simulink model "PubIfDecisionTOS_MDL"  (R2020b)
settings: configuration reference "DspaceConfig" (kept outside this file)
PostLoadFcn:
  | if any(exist('dsrtsu_mdlpostloadfcn', 'file') ~= 0), dsrtsu_mdlpostloadfcn('Execute', bdroot); end
InitFcn:
  | , if any(exist('dsmpb_private', 'file') ~= 0), dsmpb_private('dsmpb_mdlclblib', 'Init', bdroot); end,
undefined symbols (not defined in the file or in its folder): C_TOS_ACCEgoRAxletoFbumplength_m, C_TOS_ACCTargetFront_Flag, C_TOS_AEBJAPedObjDxThre_Val, C_TOS_AEBJAPedObjDyThre_Val, C_TOS_AEBJATargetSize_Val, C_TOS_AEBJAVehObjDxThre_Val, C_TOS_AEBJAVehObjDyThre_Val, C_TOS_AEBJuncPedTargetSize_Val, C_TOS_AEBLatObjDxThre_Val, C_TOS_AEBLatPedDyThre_Val, C_TOS_AEBLatTargetSize_Val, C_TOS_AEBLongTargetInEgoFront_Flag, C_TOS_axAbsGround_Parameter, C_TOS_CameraConfirmedFlag, C_TOS_CNsubjWidth, C_TOS_CurrentLaneCoreMinWidth_Val, C_TOS_CutInProb_Val_Zero, C_TOS_CutOutProb_Val_Zero, C_TOS_D2R_Val, C_TOS_DefaultValueObjectToCenterLine_dy, C_TOS_EgoCarWidth_Val, C_TOS_EgoDxRefPoint_m, C_TOS_EgoRAxletoFbumplength_m, C_TOS_HalfWidthVehicle_Con, C_TOS_HWA_CurrentLaneFlag, C_TOS_HWA_LeftLaneFlag, C_TOS_HWA_MovingDir_Vaild, C_TOS_HWA_MovState_Vaild, C_TOS_HWA_RightLaneFlag, C_TOS_LaneLineCourseErrorFront, C_TOS_LaneLineCourseErrorRear, C_TOS_MotorbikeDefaultWidth_m, C_TOS_NumberOfEffectiveTargets, C_TOS_Obj_Age_Val, C_TOS_Objdx_Constraint_Val, C_TOS_ObjectDefaultWidth_m, C_TOS_ObjInCurrentLane_Val, C_TOS_ObjInCurrentLaneValid, C_TOS_ObjInLeftLaneValid, C_TOS_ObjInRightLaneValid, C_TOS_ObjNotInCurrentLane_Val, C_TOS_ObjNotREElementType, C_TOS_ObjPredictDis_dy_ConstantVal_Zeros, C_TOS_ObjToCenterLine_ConstantVal_Zeros, C_TOS_OFMObjIDInvilad_Val, C_TOS_PIL_LatDisCons_Val_zero, C_TOS_PIL_ObjectCutInFlag_b, C_TOS_PIL_ObjectCutOutFlag_b, C_TOS_PIL_ObjLaneProb_al_Val, C_TOS_PP_ObjFusType_FC_Confirm_b, C_TOS_PP_ObjFusType_FC_FR_Confirm_b, C_TOS_PP_ObjFusType_FR_Confirm_b, C_TOS_RE_80BoolDefault_Val, C_TOS_RE_80Single181Default_Val, C_TOS_RE_80Single255Default_Val, C_TOS_RE_80Uint8Default_Val, C_TOS_RE_D2R, C_TOS_RE_D_180_Val, C_TOS_RE_InvalidObjectID_Val, C_TOS_RE_InvalidTargetChainDir_Val ... (+142)
libraries: simulink x1650, TOS_LIB x361, canfdmsglib x14
(part 64 of 69)

== stateflow chart PubIfDecisionTOS_MDL/TOS_20201112/TOS_2012080320/TOS/ACC/TOS_ACCLeftLane/ACC_LeftLane_Target/TOS_ACC_P2/ACC_P2_Targe/ACC_P2_Targe/TOS_ACC_FusionTypeConfirm/Subsystem1/TOS_ObjMovStateCfmFlow1 ==
  note: TOS_ObjMovStateCfm Coding:
      | 0: Object default moving state
      | 1：Object had been moving
      | 2: Object is moving
  (default) -> (junction 1)
  (junction 1) -> (junction 3) [order 1] : [Target_ID_K1 ~=C_TOS_OFMObjIDInvilad_Val&&...
      | Target_ID_K2 ~= C_TOS_OFMObjIDInvilad_Val]
  (junction 1) -> (junction 38) [order 2] : {
      |   TOS_ObjMovStateCfm = uint8(0);
      | }
  (junction 3) -> (junction 5)
  (junction 5) -> (junction 7) [order 1] : [Target_ID_K1 ==Target_ID_K2]
  (junction 5) -> (junction 35) [order 2] : {
      |   TOS_ObjMovStateCfm =uint8(0);
      | }
  (junction 7) -> (junction 9)
  (junction 9) -> (junction 11) [order 1] : [ObjectID ==Target_ID_K1]
  (junction 9) -> (junction 29) [order 2] : {
      |   TOS_ObjMovStateCfm = uint8(0);
      | }
  (junction 11) -> (junction 13)
  (junction 13) -> (junction 15) [order 1] : [(Target_MovState_K2 == ObjectMovingState_E.Moving||...
      | Target_MovState_K2 == ObjectMovingState_E.Stopped)&&...
      | (Target_MovState_K1 == ObjectMovingState_E.Moving||...
      | Target_MovState_K1 == ObjectMovingState_E.Stopped)||...
      |   TOS_ObjMovStateCfm == uint8(1)]
  (junction 13) -> (junction 52) [order 2]
  (junction 15) -> (junction 58) : {
      |   TOS_ObjMovStateCfm = uint8(1);
      | }
  (junction 52) -> (junction 23) [order 1] : [ObjMovState == OFM_OBJ_MOVINGSTATE_E.STOPPED||...
      | ObjMovState == OFM_OBJ_MOVINGSTATE_E.MOVING]
  (junction 52) -> (junction 27) [order 2] : {
      |   TOS_ObjMovStateCfm = uint8(0);
      | }
  (junction 23) -> (junction 54) : {
      |   TOS_ObjMovStateCfm = uint8(2);
      | }
  (junction 35) -> (junction 38)
  (junction 29) -> (junction 35)
  (junction 27) -> (junction 29)
  (junction 54) -> (junction 27)
  (junction 58) -> (junction 54)
  (junction 38) -> (junction 41)
  data: Target_ID_K1 input uint8; Target_ID_K2 input uint8; Target_MovState_K1 input Enum: ObjectMovingState_E; Target_MovState_K2 input Enum: ObjectMovingState_E; ObjMovState input Enum: OFM_OBJ_MOVINGSTATE_E; ObjectID input uint8; TOS_ObjMovStateCfm output uint8; C_TOS_OFMObjIDInvilad_Val parameter uint8

== stateflow chart PubIfDecisionTOS_MDL/TOS_20201112/TOS_2012080320/TOS/ACC/TOS_ACCLeftLane/ACC_LeftLane_Target/TOS_ACC_P2/ACC_P2_Targe/ACC_P2_Targe/TOS_ACC_ObjTypeConfirm/Subsystem1/Subsystem/TOS_ObjMovStateCfmFlow1 ==
  note: TOS_ObjMovStateCfm Coding:
      | 0: Object default moving state
      | 1：Object had been moving
      | 2: Object is moving
  (default) -> (junction 1)
  (junction 1) -> (junction 3) [order 1] : [ACC_TargetP0_ID_K1 ~=C_TOS_OFMObjIDInvilad_Val&&...
      | ACC_TargetP0_ID_K2 ~= C_TOS_OFMObjIDInvilad_Val]
  (junction 1) -> (junction 38) [order 2] : {
      |   TOS_ObjMovStateCfm = uint8(0);
      | }
  (junction 3) -> (junction 5)
  (junction 5) -> (junction 7) [order 1] : [ACC_TargetP0_ID_K1 ==ACC_TargetP0_ID_K2]
  (junction 5) -> (junction 35) [order 2] : {
      |   TOS_ObjMovStateCfm =uint8(0);
      | }
  (junction 7) -> (junction 9)
  (junction 9) -> (junction 11) [order 1] : [ObjectID ==ACC_TargetP0_ID_K1]
  (junction 9) -> (junction 29) [order 2] : {
      |   TOS_ObjMovStateCfm = uint8(0);
      | }
  (junction 11) -> (junction 13)
  (junction 13) -> (junction 15) [order 1] : [(ACC_TargetP0_MovState_K2 == ObjectMovingState_E.Moving||...
      | ACC_TargetP0_MovState_K2 == ObjectMovingState_E.Stopped)&&...
      | (ACC_TargetP0_MovState_K1 == ObjectMovingState_E.Moving||...
      | ACC_TargetP0_MovState_K1 == ObjectMovingState_E.Stopped)||...
      |   TOS_ObjMovStateCfm == uint8(1)]
  (junction 13) -> (junction 52) [order 2]
  (junction 15) -> (junction 58) : {
      |   TOS_ObjMovStateCfm = uint8(1);
      | }
  (junction 52) -> (junction 23) [order 1] : [ObjMovState == OFM_OBJ_MOVINGSTATE_E.STOPPED||...
      | ObjMovState == OFM_OBJ_MOVINGSTATE_E.MOVING]
  (junction 52) -> (junction 27) [order 2] : {
      |   TOS_ObjMovStateCfm = uint8(0);
      | }
  (junction 23) -> (junction 54) : {
      |   TOS_ObjMovStateCfm = uint8(2);
      | }
  (junction 35) -> (junction 38)
  (junction 29) -> (junction 35)
  (junction 27) -> (junction 29)
  (junction 54) -> (junction 27)
  (junction 58) -> (junction 54)
  (junction 38) -> (junction 41)
  data: ACC_TargetP0_ID_K1 input uint8; ACC_TargetP0_ID_K2 input uint8; ACC_TargetP0_MovState_K1 input Enum: ObjectMovingState_E; ACC_TargetP0_MovState_K2 input Enum: ObjectMovingState_E; ObjMovState input Enum: OFM_OBJ_MOVINGSTATE_E; ObjectID input uint8; TOS_ObjMovStateCfm output uint8; C_TOS_OFMObjIDInvilad_Val parameter uint8

== stateflow chart PubIfDecisionTOS_MDL/TOS_20201112/TOS_2012080320/TOS/ACC/TOS_ACCLeftLane/ACC_LeftLane_Target/TOS_ACC_P2/ACC_P2_Targe/ACC_P2_Targe/TOS_ACC_TargetMovingDirConfirm/Subsystem/TOS_ObjMovStateCfmFlow ==
  note: TOS_ObjMovStateCfm Coding:
      | 0: Object default moving state
      | 1：Object had been moving
      | 2: Object had been Stopped
  (default) -> (junction 1)
  (junction 1) -> (junction 3) [order 1] : [Target_ID_K1 ~=C_TOS_OFMObjIDInvilad_Val&&...
      | Target_ID_K2 ~= C_TOS_OFMObjIDInvilad_Val]
  (junction 1) -> (junction 38) [order 2] : {
      |   TOS_ObjMovStateCfm = uint8(0);
      | }
  (junction 3) -> (junction 5)
  (junction 5) -> (junction 7) [order 1] : [Target_ID_K1 ==Target_ID_K2]
  (junction 5) -> (junction 35) [order 2] : {
      |   TOS_ObjMovStateCfm =uint8(0);
      | }
  (junction 7) -> (junction 9)
  (junction 9) -> (junction 11) [order 1] : [ObjectID ==Target_ID_K1]
  (junction 9) -> (junction 29) [order 2] : {
      |   TOS_ObjMovStateCfm = uint8(0);
      | }
  (junction 11) -> (junction 13)
  (junction 13) -> (junction 15) [order 1] : [Target_MovState_K2 == ObjectMovingState_E.Moving&&...
      | Target_MovState_K1 == ObjectMovingState_E.Moving||...
      |   TOS_ObjMovStateCfm == uint8(1)]
  (junction 13) -> (junction 52) [order 2]
  (junction 15) -> (junction 58) : {
      |   TOS_ObjMovStateCfm = uint8(1);
      | }
  (junction 52) -> (junction 23) [order 1] : [Target_MovState_K2 == ObjectMovingState_E.Stopped&&...
      | Target_MovState_K1 == ObjectMovingState_E.Stopped||...
      |   TOS_ObjMovStateCfm == uint8(2)]
  (junction 52) -> (junction 27) [order 2] : {
      |   TOS_ObjMovStateCfm = uint8(0);
      | }
  (junction 23) -> (junction 54) : {
      |   TOS_ObjMovStateCfm = uint8(2);
      | }
  (junction 35) -> (junction 38)
  (junction 29) -> (junction 35)
  (junction 27) -> (junction 29)
  (junction 54) -> (junction 27)
  (junction 58) -> (junction 54)
  (junction 38) -> (junction 41)
  data: Target_ID_K1 input uint8; Target_ID_K2 input uint8; Target_MovState_K1 input Enum: ObjectMovingState_E; Target_MovState_K2 input Enum: ObjectMovingState_E; ObjMovState input Enum: OFM_OBJ_MOVINGSTATE_E; ObjectID input uint8; TOS_ObjMovStateCfm output uint8; C_TOS_OFMObjIDInvilad_Val parameter uint8

== stateflow chart PubIfDecisionTOS_MDL/TOS_20201112/TOS_2012080320/TOS/ACC/TOS_ACCLeftLane/ACC_LeftLane_Target/TOS_ACC_P4/ACC_P4_Targe/ACC_P4_Targe/TOS_ACC_FusionTypeConfirm/Subsystem1/TOS_ObjMovStateCfmFlow1 ==
  note: TOS_ObjMovStateCfm Coding:
      | 0: Object default moving state
      | 1：Object had been moving
      | 2: Object is moving
  (default) -> (junction 1)
  (junction 1) -> (junction 3) [order 1] : [Target_ID_K1 ~=C_TOS_OFMObjIDInvilad_Val&&...
      | Target_ID_K2 ~= C_TOS_OFMObjIDInvilad_Val]
  (junction 1) -> (junction 38) [order 2] : {
      |   TOS_ObjMovStateCfm = uint8(0);
      | }
  (junction 3) -> (junction 5)
  (junction 5) -> (junction 7) [order 1] : [Target_ID_K1 ==Target_ID_K2]
  (junction 5) -> (junction 35) [order 2] : {
      |   TOS_ObjMovStateCfm =uint8(0);
      | }
  (junction 7) -> (junction 9)
  (junction 9) -> (junction 11) [order 1] : [ObjectID ==Target_ID_K1]
  (junction 9) -> (junction 29) [order 2] : {
      |   TOS_ObjMovStateCfm = uint8(0);
      | }
  (junction 11) -> (junction 13)
  (junction 13) -> (junction 15) [order 1] : [(Target_MovState_K2 == ObjectMovingState_E.Moving||...
      | Target_MovState_K2 == ObjectMovingState_E.Stopped)&&...
      | (Target_MovState_K1 == ObjectMovingState_E.Moving||...
      | Target_MovState_K1 == ObjectMovingState_E.Stopped)||...
      |   TOS_ObjMovStateCfm == uint8(1)]
  (junction 13) -> (junction 52) [order 2]
  (junction 15) -> (junction 58) : {
      |   TOS_ObjMovStateCfm = uint8(1);
      | }
  (junction 52) -> (junction 23) [order 1] : [ObjMovState == OFM_OBJ_MOVINGSTATE_E.STOPPED||...
      | ObjMovState == OFM_OBJ_MOVINGSTATE_E.MOVING]
  (junction 52) -> (junction 27) [order 2] : {
      |   TOS_ObjMovStateCfm = uint8(0);
      | }
  (junction 23) -> (junction 54) : {
      |   TOS_ObjMovStateCfm = uint8(2);
      | }
  (junction 35) -> (junction 38)
  (junction 29) -> (junction 35)
  (junction 27) -> (junction 29)
  (junction 54) -> (junction 27)
  (junction 58) -> (junction 54)
  (junction 38) -> (junction 41)
  data: Target_ID_K1 input uint8; Target_ID_K2 input uint8; Target_MovState_K1 input Enum: ObjectMovingState_E; Target_MovState_K2 input Enum: ObjectMovingState_E; ObjMovState input Enum: OFM_OBJ_MOVINGSTATE_E; ObjectID input uint8; TOS_ObjMovStateCfm output uint8; C_TOS_OFMObjIDInvilad_Val parameter uint8

== stateflow chart PubIfDecisionTOS_MDL/TOS_20201112/TOS_2012080320/TOS/ACC/TOS_ACCLeftLane/ACC_LeftLane_Target/TOS_ACC_P4/ACC_P4_Targe/ACC_P4_Targe/TOS_ACC_ObjTypeConfirm/Subsystem1/Subsystem/TOS_ObjMovStateCfmFlow1 ==
  note: TOS_ObjMovStateCfm Coding:
      | 0: Object default moving state
      | 1：Object had been moving
      | 2: Object is moving
  (default) -> (junction 1)
  (junction 1) -> (junction 3) [order 1] : [ACC_TargetP0_ID_K1 ~=C_TOS_OFMObjIDInvilad_Val&&...
      | ACC_TargetP0_ID_K2 ~= C_TOS_OFMObjIDInvilad_Val]
  (junction 1) -> (junction 38) [order 2] : {
      |   TOS_ObjMovStateCfm = uint8(0);
      | }
  (junction 3) -> (junction 5)
  (junction 5) -> (junction 7) [order 1] : [ACC_TargetP0_ID_K1 ==ACC_TargetP0_ID_K2]
  (junction 5) -> (junction 35) [order 2] : {
      |   TOS_ObjMovStateCfm =uint8(0);
      | }
  (junction 7) -> (junction 9)
  (junction 9) -> (junction 11) [order 1] : [ObjectID ==ACC_TargetP0_ID_K1]
  (junction 9) -> (junction 29) [order 2] : {
      |   TOS_ObjMovStateCfm = uint8(0);
      | }
  (junction 11) -> (junction 13)
  (junction 13) -> (junction 15) [order 1] : [(ACC_TargetP0_MovState_K2 == ObjectMovingState_E.Moving||...
      | ACC_TargetP0_MovState_K2 == ObjectMovingState_E.Stopped)&&...
      | (ACC_TargetP0_MovState_K1 == ObjectMovingState_E.Moving||...
      | ACC_TargetP0_MovState_K1 == ObjectMovingState_E.Stopped)||...
      |   TOS_ObjMovStateCfm == uint8(1)]
  (junction 13) -> (junction 52) [order 2]
  (junction 15) -> (junction 58) : {
      |   TOS_ObjMovStateCfm = uint8(1);
      | }
  (junction 52) -> (junction 23) [order 1] : [ObjMovState == OFM_OBJ_MOVINGSTATE_E.STOPPED||...
      | ObjMovState == OFM_OBJ_MOVINGSTATE_E.MOVING]
  (junction 52) -> (junction 27) [order 2] : {
      |   TOS_ObjMovStateCfm = uint8(0);
      | }
  (junction 23) -> (junction 54) : {
      |   TOS_ObjMovStateCfm = uint8(2);
      | }
  (junction 35) -> (junction 38)
  (junction 29) -> (junction 35)
  (junction 27) -> (junction 29)
  (junction 54) -> (junction 27)
  (junction 58) -> (junction 54)
  (junction 38) -> (junction 41)
  data: ACC_TargetP0_ID_K1 input uint8; ACC_TargetP0_ID_K2 input uint8; ACC_TargetP0_MovState_K1 input Enum: ObjectMovingState_E; ACC_TargetP0_MovState_K2 input Enum: ObjectMovingState_E; ObjMovState input Enum: OFM_OBJ_MOVINGSTATE_E; ObjectID input uint8; TOS_ObjMovStateCfm output uint8; C_TOS_OFMObjIDInvilad_Val parameter uint8

== stateflow chart PubIfDecisionTOS_MDL/TOS_20201112/TOS_2012080320/TOS/ACC/TOS_ACCLeftLane/ACC_LeftLane_Target/TOS_ACC_P4/ACC_P4_Targe/ACC_P4_Targe/TOS_ACC_TargetMovingDirConfirm/Subsystem/TOS_ObjMovStateCfmFlow ==
  note: TOS_ObjMovStateCfm Coding:
      | 0: Object default moving state
      | 1：Object had been moving
      | 2: Object had been Stopped
  (default) -> (junction 1)
  (junction 1) -> (junction 3) [order 1] : [Target_ID_K1 ~=C_TOS_OFMObjIDInvilad_Val&&...
      | Target_ID_K2 ~= C_TOS_OFMObjIDInvilad_Val]
  (junction 1) -> (junction 38) [order 2] : {
      |   TOS_ObjMovStateCfm = uint8(0);
      | }
  (junction 3) -> (junction 5)
  (junction 5) -> (junction 7) [order 1] : [Target_ID_K1 ==Target_ID_K2]
  (junction 5) -> (junction 35) [order 2] : {
      |   TOS_ObjMovStateCfm =uint8(0);
      | }
  (junction 7) -> (junction 9)
  (junction 9) -> (junction 11) [order 1] : [ObjectID ==Target_ID_K1]
  (junction 9) -> (junction 29) [order 2] : {
      |   TOS_ObjMovStateCfm = uint8(0);
      | }
  (junction 11) -> (junction 13)
  (junction 13) -> (junction 15) [order 1] : [Target_MovState_K2 == ObjectMovingState_E.Moving&&...
      | Target_MovState_K1 == ObjectMovingState_E.Moving||...
      |   TOS_ObjMovStateCfm == uint8(1)]
  (junction 13) -> (junction 52) [order 2]
  (junction 15) -> (junction 58) : {
      |   TOS_ObjMovStateCfm = uint8(1);
      | }
  (junction 52) -> (junction 23) [order 1] : [Target_MovState_K2 == ObjectMovingState_E.Stopped&&...
      | Target_MovState_K1 == ObjectMovingState_E.Stopped||...
      |   TOS_ObjMovStateCfm == uint8(2)]
  (junction 52) -> (junction 27) [order 2] : {
      |   TOS_ObjMovStateCfm = uint8(0);
      | }
  (junction 23) -> (junction 54) : {
      |   TOS_ObjMovStateCfm = uint8(2);
      | }
  (junction 35) -> (junction 38)
  (junction 29) -> (junction 35)
  (junction 27) -> (junction 29)
  (junction 54) -> (junction 27)
  (junction 58) -> (junction 54)
  (junction 38) -> (junction 41)
  data: Target_ID_K1 input uint8; Target_ID_K2 input uint8; Target_MovState_K1 input Enum: ObjectMovingState_E; Target_MovState_K2 input Enum: ObjectMovingState_E; ObjMovState input Enum: OFM_OBJ_MOVINGSTATE_E; ObjectID input uint8; TOS_ObjMovStateCfm output uint8; C_TOS_OFMObjIDInvilad_Val parameter uint8

== matlab function PubIfDecisionTOS_MDL/TOS_20201112/TOS_2012080320/TOS/ACC/TOS_ACCLeftLane/MATLAB Function1 ==
  data: Object_Dx input; Object_ID input; Dx1stNearestObjIndex output; Dx2edNearestObjIndex output; Dx1stNearestObjID output; Dx2edNearestObjID output; ConditionJudge input; TOS_ACC_P2_P4_TargetPre_Confirm_FiltFlag input; Object_Num input

%%%%ObjDisIndex按Dx从小到大的总排序
%%%%%%%%ObjectID按Dx从小到大的总排序
function [Dx1stNearestObjIndex,Dx2edNearestObjIndex,Dx1stNearestObjID,Dx2edNearestObjID]   = MinMax(Object_Dx,Object_ID,ConditionJudge,TOS_ACC_P2_P4_TargetPre_Confirm_FiltFlag,Object_Num)
Dx = Object_Dx;
ID = Object_ID;
for i=int32(1):int32(Object_Num)
    
    if (ID(i) == uint8(0))||(ConditionJudge(i) == false)||(Dx(i) < single(0))||(TOS_ACC_P2_P4_TargetPre_Confirm_FiltFlag(i) == false)%%%%%本车道/前方/非0目标
       Dx(i) = single(255);
    end
end

[MinDx1st,MinIndex1st] = min(Dx);
if (MinDx1st > single(250))
   Dx1stNearestObjIndex = uint8(0);
   Dx1stNearestObjID = uint8(0); 
   Dx2edNearestObjIndex = uint8(0);
   Dx2edNearestObjID = uint8(0);
else
    Dx(MinIndex1st) = single(255);
    [MinDx2ed,MinIndex2ed] = min(Dx);
    Dx1stNearestObjIndex = uint8(MinIndex1st);
   Dx1stNearestObjID = uint8(ID(MinIndex1st)); 
   
   if (MinDx2ed > single(250))
     Dx2edNearestObjIndex = uint8(0);
     Dx2edNearestObjID = uint8(0);
   else
     Dx2edNearestObjIndex = uint8(MinIndex2ed);
     Dx2edNearestObjID = uint8(ID(MinIndex2ed));
   end
   

end
end

== stateflow chart PubIfDecisionTOS_MDL/TOS_20201112/TOS_2012080320/TOS/ACC/TOS_ACCRightLane/ACCTargetPO35Infor/TOS_ACCPO3TargetInfor ==
  (default) -> (junction 1)
  (junction 1) -> (junction 3) [order 1] : [TOS_ACCPO3TargetIndex ~= uint8(0)]
  (junction 1) -> (junction 7) [order 2] : {TOS_ACCPO3TargetInfo.IDP3= uint8(0);
      | TOS_ACCPO3TargetInfo.dxP3=single(255);
      | TOS_ACCPO3TargetInfo.vxRelP3= single(0);
      | TOS_ACCPO3TargetInfo.axAbsGroundP3=single(0);
      | TOS_ACCPO3TargetInfo.rangeP3=single(0);
      | TOS_ACCPO3TargetInfo.targetExistP3= boolean(0);
      | TOS_ACCPO3TargetInfo.fu_typeP3= uint8(0);
      | TOS_ACCPO3TargetInfo.ObjMovingStateP3= uint8(0);
      | TOS_ACCPO3TargetInfo.ObjTypeP3= uint8(0);
      | TOS_ACCPO3TargetInfo.ObjDYP3=single(255);
      | TOS_ACCPO3TargetInfo.P3HeadingAngle=single(0);
      | TOS_ACCPO3TargetInfo.P3CutinProb= single(0);
      | }
  (junction 3) -> (junction 5) : {
      | TOS_ACCPO3TargetInfo.IDP3=OFM_SignalVerification.Object_ID[TOS_ACCPO3TargetIndex- uint8(1)];
      | TOS_ACCPO3TargetInfo.dxP3=OFM_SignalVerification.Object_DX[TOS_ACCPO3TargetIndex-uint8(1)];
      | TOS_ACCPO3TargetInfo.vxRelP3=OFM_SignalVerification.Object_VX[TOS_ACCPO3TargetIndex-uint8(1)];
      | TOS_ACCPO3TargetInfo.axAbsGroundP3=TOS_AddAttributes.PP_axAbsGround[TOS_ACCPO3TargetIndex-uint8(1)];
      | TOS_ACCPO3TargetInfo.rangeP3=TOS_AddAttributes.PP_ObjToEgoCarFrontbump[TOS_ACCPO3TargetIndex-uint8(1)];
      | TOS_ACCPO3TargetInfo.targetExistP3=boolean(1);
      | TOS_ACCPO3TargetInfo.fu_typeP3=OFM_SignalVerification.Object_Fus_Type[TOS_ACCPO3TargetIndex-uint8(1)];
      | TOS_ACCPO3TargetInfo.ObjMovingStateP3=TOS_AddAttributes.PP_MovingStateSignalProcessing[TOS_ACCPO3TargetIndex-uint8(1)];
      | TOS_ACCPO3TargetInfo.ObjTypeP3=OFM_SignalVerification.Object_Type[TOS_ACCPO3TargetIndex-uint8(1)];
      | TOS_ACCPO3TargetInfo.ObjDYP3=OFM_SignalVerification.Object_DY[TOS_ACCPO3TargetIndex-uint8(1)];
      | TOS_ACCPO3TargetInfo.P3HeadingAngle=OFM_SignalVerification.Object_HeadingAngle[TOS_ACCPO3TargetIndex-uint8(1)];
      | TOS_ACCPO3TargetInfo.P3CutinProb =TOS_ProbInLaneCalculat.PIL_CutinProb[TOS_ACCPO3TargetIndex-uint8(1)];
      | }
  (junction 5) -> (junction 7)
  (junction 7) -> (junction 11)
  data: OFM_SignalVerification input Bus: OFM_OBJ_BUS; TOS_AddAttributes input Bus: TOS_AddAttributes_BUS; TOS_ProbInLaneCalculat input Bus: PIL_ProbInLaneCalculat_BUS; TOS_ACCPO3TargetIndex input uint8; TOS_ACCPO3TargetInfo output Bus: TOS_ACCP3_BUS =0

== stateflow chart PubIfDecisionTOS_MDL/TOS_20201112/TOS_2012080320/TOS/ACC/TOS_ACCRightLane/ACCTargetPO35Infor/TOS_ACCPO5TargetInfor ==
  (default) -> (junction 1)
  (junction 1) -> (junction 3) [order 1] : [TOS_ACCPO5TargetIndex ~= uint8(0)]
  (junction 1) -> (junction 7) [order 2] : {
      | TOS_ACCPO5TargetInfo.dyP5= uint8(0);
      | TOS_ACCPO5TargetInfo.dxP5=single(255);
      | TOS_ACCPO5TargetInfo.targetExistP5= boolean(1);
      | TOS_ACCPO5TargetInfo.ObjTypeP5= uint8(0);
      | }
  (junction 3) -> (junction 5) : {
      | TOS_ACCPO5TargetInfo.dyP5                     =OFM_SignalVerification.Object_DY[TOS_ACCPO5TargetIndex-uint8(1)];
      | TOS_ACCPO5TargetInfo.dxP5                     =OFM_SignalVerification.Object_DX[TOS_ACCPO5TargetIndex-uint8(1)];
      | TOS_ACCPO5TargetInfo.targetExistP5        =boolean(1);
      | TOS_ACCPO5TargetInfo.ObjTypeP5           =OFM_SignalVerification.Object_Type[TOS_ACCPO5TargetIndex-uint8(1)];
      | }
  (junction 5) -> (junction 7)
  (junction 7) -> (junction 11)
  data: OFM_SignalVerification input Bus: OFM_OBJ_BUS; TOS_ACCPO5TargetIndex input uint8; TOS_ACCPO5TargetInfo output Bus: TOS_ACCP5_BUS =0

== stateflow chart PubIfDecisionTOS_MDL/TOS_20201112/TOS_2012080320/TOS/ACC/TOS_ACCRightLane/ACC_LeftLane_Target/TOS_ACC_P3/ACC_P3_Targe/ACC_P3_Targe/TOS_ACC_FusionTypeConfirm/Subsystem1/TOS_ObjMovStateCfmFlow1 ==
  note: TOS_ObjMovStateCfm Coding:
      | 0: Object default moving state
      | 1：Object had been moving
      | 2: Object is moving
  (default) -> (junction 1)
  (junction 1) -> (junction 3) [order 1] : [Target_ID_K1 ~=C_TOS_OFMObjIDInvilad_Val&&...
      | Target_ID_K2 ~= C_TOS_OFMObjIDInvilad_Val]
  (junction 1) -> (junction 38) [order 2] : {
      |   TOS_ObjMovStateCfm = uint8(0);
      | }
  (junction 3) -> (junction 5)
  (junction 5) -> (junction 7) [order 1] : [Target_ID_K1 ==Target_ID_K2]
  (junction 5) -> (junction 35) [order 2] : {
      |   TOS_ObjMovStateCfm =uint8(0);
      | }
  (junction 7) -> (junction 9)
  (junction 9) -> (junction 11) [order 1] : [ObjectID ==Target_ID_K1]
  (junction 9) -> (junction 29) [order 2] : {
      |   TOS_ObjMovStateCfm = uint8(0);
      | }
  (junction 11) -> (junction 13)
  (junction 13) -> (junction 15) [order 1] : [(Target_MovState_K2 == ObjectMovingState_E.Moving||...
      | Target_MovState_K2 == ObjectMovingState_E.Stopped)&&...
      | (Target_MovState_K1 == ObjectMovingState_E.Moving||...
      | Target_MovState_K1 == ObjectMovingState_E.Stopped)||...
      |   TOS_ObjMovStateCfm == uint8(1)]
  (junction 13) -> (junction 52) [order 2]
  (junction 15) -> (junction 58) : {
      |   TOS_ObjMovStateCfm = uint8(1);
      | }
  (junction 52) -> (junction 23) [order 1] : [ObjMovState == OFM_OBJ_MOVINGSTATE_E.STOPPED||...
      | ObjMovState == OFM_OBJ_MOVINGSTATE_E.MOVING]
  (junction 52) -> (junction 27) [order 2] : {
      |   TOS_ObjMovStateCfm = uint8(0);
      | }
  (junction 23) -> (junction 54) : {
      |   TOS_ObjMovStateCfm = uint8(2);
      | }
  (junction 35) -> (junction 38)
  (junction 29) -> (junction 35)
  (junction 27) -> (junction 29)
  (junction 54) -> (junction 27)
  (junction 58) -> (junction 54)
  (junction 38) -> (junction 41)
  data: Target_ID_K1 input uint8; Target_ID_K2 input uint8; Target_MovState_K1 input Enum: ObjectMovingState_E; Target_MovState_K2 input Enum: ObjectMovingState_E; ObjMovState input Enum: OFM_OBJ_MOVINGSTATE_E; ObjectID input uint8; TOS_ObjMovStateCfm output uint8; C_TOS_OFMObjIDInvilad_Val parameter uint8

== stateflow chart PubIfDecisionTOS_MDL/TOS_20201112/TOS_2012080320/TOS/ACC/TOS_ACCRightLane/ACC_LeftLane_Target/TOS_ACC_P3/ACC_P3_Targe/ACC_P3_Targe/TOS_ACC_ObjTypeConfirm/Subsystem1/Subsystem/TOS_ObjMovStateCfmFlow1 ==
  note: TOS_ObjMovStateCfm Coding:
      | 0: Object default moving state
      | 1：Object had been moving
      | 2: Object is moving
  (default) -> (junction 1)
  (junction 1) -> (junction 3) [order 1] : [ACC_TargetP0_ID_K1 ~=C_TOS_OFMObjIDInvilad_Val&&...
      | ACC_TargetP0_ID_K2 ~= C_TOS_OFMObjIDInvilad_Val]
  (junction 1) -> (junction 38) [order 2] : {
      |   TOS_ObjMovStateCfm = uint8(0);
      | }
  (junction 3) -> (junction 5)
  (junction 5) -> (junction 7) [order 1] : [ACC_TargetP0_ID_K1 ==ACC_TargetP0_ID_K2]
  (junction 5) -> (junction 35) [order 2] : {
      |   TOS_ObjMovStateCfm =uint8(0);
      | }
  (junction 7) -> (junction 9)
  (junction 9) -> (junction 11) [order 1] : [ObjectID ==ACC_TargetP0_ID_K1]
  (junction 9) -> (junction 29) [order 2] : {
      |   TOS_ObjMovStateCfm = uint8(0);
      | }
  (junction 11) -> (junction 13)
  (junction 13) -> (junction 15) [order 1] : [(ACC_TargetP0_MovState_K2 == ObjectMovingState_E.Moving||...
      | ACC_TargetP0_MovState_K2 == ObjectMovingState_E.Stopped)&&...
      | (ACC_TargetP0_MovState_K1 == ObjectMovingState_E.Moving||...
      | ACC_TargetP0_MovState_K1 == ObjectMovingState_E.Stopped)||...
      |   TOS_ObjMovStateCfm == uint8(1)]
  (junction 13) -> (junction 52) [order 2]
  (junction 15) -> (junction 58) : {
      |   TOS_ObjMovStateCfm = uint8(1);
      | }
  (junction 52) -> (junction 23) [order 1] : [ObjMovState == OFM_OBJ_MOVINGSTATE_E.STOPPED||...
      | ObjMovState == OFM_OBJ_MOVINGSTATE_E.MOVING]
  (junction 52) -> (junction 27) [order 2] : {
      |   TOS_ObjMovStateCfm = uint8(0);
      | }
  (junction 23) -> (junction 54) : {
      |   TOS_ObjMovStateCfm = uint8(2);
      | }
  (junction 35) -> (junction 38)
  (junction 29) -> (junction 35)
  (junction 27) -> (junction 29)
  (junction 54) -> (junction 27)
  (junction 58) -> (junction 54)
  (junction 38) -> (junction 41)
  data: ACC_TargetP0_ID_K1 input uint8; ACC_TargetP0_ID_K2 input uint8; ACC_TargetP0_MovState_K1 input Enum: ObjectMovingState_E; ACC_TargetP0_MovState_K2 input Enum: ObjectMovingState_E; ObjMovState input Enum: OFM_OBJ_MOVINGSTATE_E; ObjectID input uint8; TOS_ObjMovStateCfm output uint8; C_TOS_OFMObjIDInvilad_Val parameter uint8

== stateflow chart PubIfDecisionTOS_MDL/TOS_20201112/TOS_2012080320/TOS/ACC/TOS_ACCRightLane/ACC_LeftLane_Target/TOS_ACC_P3/ACC_P3_Targe/ACC_P3_Targe/TOS_ACC_TargetMovingDirConfirm/Subsystem/TOS_ObjMovStateCfmFlow ==
  note: TOS_ObjMovStateCfm Coding:
      | 0: Object default moving state
      | 1：Object had been moving
      | 2: Object had been Stopped
  (default) -> (junction 1)
  (junction 1) -> (junction 3) [order 1] : [Target_ID_K1 ~=C_TOS_OFMObjIDInvilad_Val&&...
      | Target_ID_K2 ~= C_TOS_OFMObjIDInvilad_Val]
  (junction 1) -> (junction 38) [order 2] : {
      |   TOS_ObjMovStateCfm = uint8(0);
      | }
  (junction 3) -> (junction 5)
  (junction 5) -> (junction 7) [order 1] : [Target_ID_K1 ==Target_ID_K2]
  (junction 5) -> (junction 35) [order 2] : {
      |   TOS_ObjMovStateCfm =uint8(0);
      | }
  (junction 7) -> (junction 9)
  (junction 9) -> (junction 11) [order 1] : [ObjectID ==Target_ID_K1]
  (junction 9) -> (junction 29) [order 2] : {
      |   TOS_ObjMovStateCfm = uint8(0);
      | }
  (junction 11) -> (junction 13)
  (junction 13) -> (junction 15) [order 1] : [Target_MovState_K2 == ObjectMovingState_E.Moving&&...
      | Target_MovState_K1 == ObjectMovingState_E.Moving||...
      |   TOS_ObjMovStateCfm == uint8(1)]
  (junction 13) -> (junction 52) [order 2]
  (junction 15) -> (junction 58) : {
      |   TOS_ObjMovStateCfm = uint8(1);
      | }
  (junction 52) -> (junction 23) [order 1] : [Target_MovState_K2 == ObjectMovingState_E.Stopped&&...
      | Target_MovState_K1 == ObjectMovingState_E.Stopped||...
      |   TOS_ObjMovStateCfm == uint8(2)]
  (junction 52) -> (junction 27) [order 2] : {
      |   TOS_ObjMovStateCfm = uint8(0);
      | }
  (junction 23) -> (junction 54) : {
      |   TOS_ObjMovStateCfm = uint8(2);
      | }
  (junction 35) -> (junction 38)
  (junction 29) -> (junction 35)
  (junction 27) -> (junction 29)
  (junction 54) -> (junction 27)
  (junction 58) -> (junction 54)
  (junction 38) -> (junction 41)
  data: Target_ID_K1 input uint8; Target_ID_K2 input uint8; Target_MovState_K1 input Enum: ObjectMovingState_E; Target_MovState_K2 input Enum: ObjectMovingState_E; ObjMovState input Enum: OFM_OBJ_MOVINGSTATE_E; ObjectID input uint8; TOS_ObjMovStateCfm output uint8; C_TOS_OFMObjIDInvilad_Val parameter uint8

== stateflow chart PubIfDecisionTOS_MDL/TOS_20201112/TOS_2012080320/TOS/ACC/TOS_ACCRightLane/ACC_LeftLane_Target/TOS_ACC_P5/ACC_P5_Targe/ACC_P5_Targe/TOS_ACC_FusionTypeConfirm/Subsystem1/TOS_ObjMovStateCfmFlow1 ==
  note: TOS_ObjMovStateCfm Coding:
      | 0: Object default moving state
      | 1：Object had been moving
      | 2: Object is moving
  (default) -> (junction 1)
  (junction 1) -> (junction 3) [order 1] : [Target_ID_K1 ~=C_TOS_OFMObjIDInvilad_Val&&...
      | Target_ID_K2 ~= C_TOS_OFMObjIDInvilad_Val]
  (junction 1) -> (junction 38) [order 2] : {
      |   TOS_ObjMovStateCfm = uint8(0);
      | }
  (junction 3) -> (junction 5)
  (junction 5) -> (junction 7) [order 1] : [Target_ID_K1 ==Target_ID_K2]
  (junction 5) -> (junction 35) [order 2] : {
      |   TOS_ObjMovStateCfm =uint8(0);
      | }
  (junction 7) -> (junction 9)
  (junction 9) -> (junction 11) [order 1] : [ObjectID ==Target_ID_K1]
  (junction 9) -> (junction 29) [order 2] : {
      |   TOS_ObjMovStateCfm = uint8(0);
      | }
  (junction 11) -> (junction 13)
  (junction 13) -> (junction 15) [order 1] : [(Target_MovState_K2 == ObjectMovingState_E.Moving||...
      | Target_MovState_K2 == ObjectMovingState_E.Stopped)&&...
      | (Target_MovState_K1 == ObjectMovingState_E.Moving||...
      | Target_MovState_K1 == ObjectMovingState_E.Stopped)||...
      |   TOS_ObjMovStateCfm == uint8(1)]
  (junction 13) -> (junction 52) [order 2]
  (junction 15) -> (junction 58) : {
      |   TOS_ObjMovStateCfm = uint8(1);
      | }
  (junction 52) -> (junction 23) [order 1] : [ObjMovState == OFM_OBJ_MOVINGSTATE_E.STOPPED||...
      | ObjMovState == OFM_OBJ_MOVINGSTATE_E.MOVING]
  (junction 52) -> (junction 27) [order 2] : {
      |   TOS_ObjMovStateCfm = uint8(0);
      | }
  (junction 23) -> (junction 54) : {
      |   TOS_ObjMovStateCfm = uint8(2);
      | }
  (junction 35) -> (junction 38)
  (junction 29) -> (junction 35)
  (junction 27) -> (junction 29)
  (junction 54) -> (junction 27)
  (junction 58) -> (junction 54)
  (junction 38) -> (junction 41)
  data: Target_ID_K1 input uint8; Target_ID_K2 input uint8; Target_MovState_K1 input Enum: ObjectMovingState_E; Target_MovState_K2 input Enum: ObjectMovingState_E; ObjMovState input Enum: OFM_OBJ_MOVINGSTATE_E; ObjectID input uint8; TOS_ObjMovStateCfm output uint8; C_TOS_OFMObjIDInvilad_Val parameter uint8

== stateflow chart PubIfDecisionTOS_MDL/TOS_20201112/TOS_2012080320/TOS/ACC/TOS_ACCRightLane/ACC_LeftLane_Target/TOS_ACC_P5/ACC_P5_Targe/ACC_P5_Targe/TOS_ACC_ObjTypeConfirm/Subsystem1/Subsystem/TOS_ObjMovStateCfmFlow1 ==
  note: TOS_ObjMovStateCfm Coding:
      | 0: Object default moving state
      | 1：Object had been moving
      | 2: Object is moving
  (default) -> (junction 1)
  (junction 1) -> (junction 3) [order 1] : [ACC_TargetP0_ID_K1 ~=C_TOS_OFMObjIDInvilad_Val&&...
      | ACC_TargetP0_ID_K2 ~= C_TOS_OFMObjIDInvilad_Val]
  (junction 1) -> (junction 38) [order 2] : {
      |   TOS_ObjMovStateCfm = uint8(0);
      | }
  (junction 3) -> (junction 5)
  (junction 5) -> (junction 7) [order 1] : [ACC_TargetP0_ID_K1 ==ACC_TargetP0_ID_K2]
  (junction 5) -> (junction 35) [order 2] : {
      |   TOS_ObjMovStateCfm =uint8(0);
      | }
  (junction 7) -> (junction 9)
  (junction 9) -> (junction 11) [order 1] : [ObjectID ==ACC_TargetP0_ID_K1]
  (junction 9) -> (junction 29) [order 2] : {
      |   TOS_ObjMovStateCfm = uint8(0);
      | }
  (junction 11) -> (junction 13)
  (junction 13) -> (junction 15) [order 1] : [(ACC_TargetP0_MovState_K2 == ObjectMovingState_E.Moving||...
      | ACC_TargetP0_MovState_K2 == ObjectMovingState_E.Stopped)&&...
      | (ACC_TargetP0_MovState_K1 == ObjectMovingState_E.Moving||...
      | ACC_TargetP0_MovState_K1 == ObjectMovingState_E.Stopped)||...
      |   TOS_ObjMovStateCfm == uint8(1)]
  (junction 13) -> (junction 52) [order 2]
  (junction 15) -> (junction 58) : {
      |   TOS_ObjMovStateCfm = uint8(1);
      | }
  (junction 52) -> (junction 23) [order 1] : [ObjMovState == OFM_OBJ_MOVINGSTATE_E.STOPPED||...
      | ObjMovState == OFM_OBJ_MOVINGSTATE_E.MOVING]
  (junction 52) -> (junction 27) [order 2] : {
      |   TOS_ObjMovStateCfm = uint8(0);
      | }
  (junction 23) -> (junction 54) : {
      |   TOS_ObjMovStateCfm = uint8(2);
      | }
  (junction 35) -> (junction 38)
  (junction 29) -> (junction 35)
  (junction 27) -> (junction 29)
  (junction 54) -> (junction 27)
  (junction 58) -> (junction 54)
  (junction 38) -> (junction 41)
  data: ACC_TargetP0_ID_K1 input uint8; ACC_TargetP0_ID_K2 input uint8; ACC_TargetP0_MovState_K1 input Enum: ObjectMovingState_E; ACC_TargetP0_MovState_K2 input Enum: ObjectMovingState_E; ObjMovState input Enum: OFM_OBJ_MOVINGSTATE_E; ObjectID input uint8; TOS_ObjMovStateCfm output uint8; C_TOS_OFMObjIDInvilad_Val parameter uint8

== stateflow chart PubIfDecisionTOS_MDL/TOS_20201112/TOS_2012080320/TOS/ACC/TOS_ACCRightLane/ACC_LeftLane_Target/TOS_ACC_P5/ACC_P5_Targe/ACC_P5_Targe/TOS_ACC_TargetMovingDirConfirm/Subsystem/TOS_ObjMovStateCfmFlow ==
  note: TOS_ObjMovStateCfm Coding:
      | 0: Object default moving state
      | 1：Object had been moving
      | 2: Object had been Stopped
  (default) -> (junction 1)
  (junction 1) -> (junction 3) [order 1] : [Target_ID_K1 ~=C_TOS_OFMObjIDInvilad_Val&&...
      | Target_ID_K2 ~= C_TOS_OFMObjIDInvilad_Val]
  (junction 1) -> (junction 38) [order 2] : {
      |   TOS_ObjMovStateCfm = uint8(0);
      | }
  (junction 3) -> (junction 5)
  (junction 5) -> (junction 7) [order 1] : [Target_ID_K1 ==Target_ID_K2]
  (junction 5) -> (junction 35) [order 2] : {
      |   TOS_ObjMovStateCfm =uint8(0);
      | }
  (junction 7) -> (junction 9)
  (junction 9) -> (junction 11) [order 1] : [ObjectID ==Target_ID_K1]
  (junction 9) -> (junction 29) [order 2] : {
      |   TOS_ObjMovStateCfm = uint8(0);
      | }
  (junction 11) -> (junction 13)
  (junction 13) -> (junction 15) [order 1] : [Target_MovState_K2 == ObjectMovingState_E.Moving&&...
      | Target_MovState_K1 == ObjectMovingState_E.Moving||...
      |   TOS_ObjMovStateCfm == uint8(1)]
  (junction 13) -> (junction 52) [order 2]
  (junction 15) -> (junction 58) : {
      |   TOS_ObjMovStateCfm = uint8(1);
      | }
  (junction 52) -> (junction 23) [order 1] : [Target_MovState_K2 == ObjectMovingState_E.Stopped&&...
      | Target_MovState_K1 == ObjectMovingState_E.Stopped||...
      |   TOS_ObjMovStateCfm == uint8(2)]
  (junction 52) -> (junction 27) [order 2] : {
      |   TOS_ObjMovStateCfm = uint8(0);
      | }
  (junction 23) -> (junction 54) : {
      |   TOS_ObjMovStateCfm = uint8(2);
      | }
  (junction 35) -> (junction 38)
  (junction 29) -> (junction 35)
  (junction 27) -> (junction 29)
  (junction 54) -> (junction 27)
  (junction 58) -> (junction 54)
  (junction 38) -> (junction 41)
  data: Target_ID_K1 input uint8; Target_ID_K2 input uint8; Target_MovState_K1 input Enum: ObjectMovingState_E; Target_MovState_K2 input Enum: ObjectMovingState_E; ObjMovState input Enum: OFM_OBJ_MOVINGSTATE_E; ObjectID input uint8; TOS_ObjMovStateCfm output uint8; C_TOS_OFMObjIDInvilad_Val parameter uint8

== matlab function PubIfDecisionTOS_MDL/TOS_20201112/TOS_2012080320/TOS/ACC/TOS_ACCRightLane/MATLAB Function1 ==
  data: Object_Dx input; Object_ID input; Dx1stNearestObjIndex output; Dx2edNearestObjIndex output; Dx1stNearestObjID output; Dx2edNearestObjID output; ConditionJudge input; TargetFusionTypeFlag input; Object_Num input

%%%%ObjDisIndex按Dx从小到大的总排序
%%%%%%%%ObjectID按Dx从小到大的总排序
function [Dx1stNearestObjIndex,Dx2edNearestObjIndex,Dx1stNearestObjID,Dx2edNearestObjID]   = MinMax(Object_Dx,Object_ID,ConditionJudge,TargetFusionTypeFlag,Object_Num)
Dx = Object_Dx;
ID = Object_ID;
for i=int32(1):int32(Object_Num)
    
    if (ID(i) == uint8(0))||(ConditionJudge(i) == false)||(Dx(i) < single(0))||(TargetFusionTypeFlag(i) == false)%%%%%本车道/前方/非0目标
       Dx(i) = single(255);
    end
end

[MinDx1st,MinIndex1st] = min(Dx);
if (MinDx1st > single(250))
   Dx1stNearestObjIndex = uint8(0);
   Dx1stNearestObjID = uint8(0); 
   Dx2edNearestObjIndex = uint8(0);
   Dx2edNearestObjID = uint8(0);
else
    Dx(MinIndex1st) = single(255);
    [MinDx2ed,MinIndex2ed] = min(Dx);
    Dx1stNearestObjIndex = uint8(MinIndex1st);
   Dx1stNearestObjID = uint8(ID(MinIndex1st)); 
   
   if (MinDx2ed > single(250))
     Dx2edNearestObjIndex = uint8(0);
     Dx2edNearestObjID = uint8(0);
   else
     Dx2edNearestObjIndex = uint8(MinIndex2ed);
     Dx2edNearestObjID = uint8(ID(MinIndex2ed));
   end
   

end
end

== matlab function PubIfDecisionTOS_MDL/TOS_20201112/TOS_2012080320/TOS/AEB/TOS_AEBJunct1105/AEBJuncTargetIndex/MATLAB Function ==
  data: Distance input; Object_Num input; ObjDisIndex output
function ObjDisIndex  = fcn(Distance,Object_Num)
ObjNum=80;
ObjDisIndex=uint8(zeros(ObjNum,1));
DxDy=Distance;
MidIndex=1:1:ObjNum;
for i=1:Object_Num
    ObjDisIndex(i)=MidIndex(i);
    t_dis=DxDy(i);
    if i<Object_Num-1
        for j=(i+1):Object_Num
            if DxDy(j)<t_dis
                temp_index=ObjDisIndex(i);
                temp_dis=t_dis;
                ObjDisIndex(i)=MidIndex(j);
                DxDy(i)=DxDy(j);
                t_dis=DxDy(j);
                MidIndex(j)=temp_index;
                DxDy(j)=temp_dis;
            end
            
            if DxDy(i) >= single(250)     
                ObjDisIndex(i)=uint8(0); 
            end           
   
        end
    else
        if i~=Object_Num
            if DxDy(Object_Num)<t_dis
                temp_index=ObjDisIndex(i);
                temp_dis=t_dis;
                ObjDisIndex(i)=MidIndex(Object_Num);
                DxDy(i)=DxDy(Object_Num);
                MidIndex(Object_Num)=temp_index;
                DxDy(Object_Num)=temp_dis;
            else
                MidIndex(Object_Num)=MidIndex(Object_Num);
                DxDy(Object_Num)=DxDy(Object_Num);
            end
            
            if DxDy(i) >= single(250)     
                ObjDisIndex(i)=uint8(0); 
            end       
            
        end
    end

end

== matlab function PubIfDecisionTOS_MDL/TOS_20201112/TOS_2012080320/TOS/AEB/TOS_AEBJunct1105/AEBJuncTargetIndex/MATLAB Function1 ==
  data: Object_Num input; Distance input; ObjDisIndex output
function ObjDisIndex  = fcn(Object_Num,Distance)
ObjNum=80;
ObjDisIndex=uint8(zeros(ObjNum,1));
DxDy=Distance;
MidIndex=1:1:ObjNum;
for i=1:Object_Num
    ObjDisIndex(i)=MidIndex(i);
    t_dis=DxDy(i);
    if i<Object_Num-1
        for j=(i+1):Object_Num
            if DxDy(j)<t_dis
                temp_index=ObjDisIndex(i);
                temp_dis=t_dis;
                ObjDisIndex(i)=MidIndex(j);
                DxDy(i)=DxDy(j);
                t_dis=DxDy(j);
                MidIndex(j)=temp_index;
                DxDy(j)=temp_dis;
            end
            
            if DxDy(i) >= single(250)     
                ObjDisIndex(i)=uint8(0); 
            end           
   
        end
    else
        if i~=Object_Num
            if DxDy(Object_Num)<t_dis
                temp_index=ObjDisIndex(i);
                temp_dis=t_dis;
                ObjDisIndex(i)=MidIndex(Object_Num);
                DxDy(i)=DxDy(Object_Num);
                MidIndex(Object_Num)=temp_index;
                DxDy(Object_Num)=temp_dis;
            else
                MidIndex(Object_Num)=MidIndex(Object_Num);
                DxDy(Object_Num)=DxDy(Object_Num);
            end
            
            if DxDy(i) >= single(250)     
                ObjDisIndex(i)=uint8(0); 
            end       
            
        end
    end

end

== stateflow chart PubIfDecisionTOS_MDL/TOS_20201112/TOS_2012080320/TOS/AEB/TOS_AEBJunct1105/AEBJunc_Object_Condition/AEBJA_TargetCondition/TOS_AEBJunc_TargetsCondition/AEBJunc_PedTargetCondition/Chart ==
  state AEBJuncSameTargetIDJudge [function]
    (default) -> (junction 70) : {
        | i = uint8(1);
        | AEBJunc_SameTarget = false;
        | }
    (junction 70) -> (junction 81) [order 1] : [i<=C_TOS_AEBJuncPedTargetSize_Val]
    (junction 86) -> (junction 70)
    (junction 70) -> (junction 83) [order 2]
    (junction 81) -> (junction 77)
    (junction 77) -> (junction 78) [order 1] : [AEBJunc_Target_ObjectID_K1(i) == Object_ID]
    (junction 77) -> (junction 74) [order 2] : %donothing
    (junction 78) -> (junction 72) : {
        | AEBJunc_SameTarget = true;
        | }
    (junction 72) -> (junction 74)
    (junction 74) -> (junction 86) : {i = i+1;}
  (default) -> (junction 1)
  (junction 1) -> (junction 3) [order 1] : [AEBJunc_TargetCondition == true]
  (junction 1) -> (junction 97) [order 2] : {
      | TOS_AEBJunc_TargetsDx = single(255);
      | }
  (junction 3) -> (junction 88) : {
      | AEBJuncSameTargetIDJudge();
      | }
  (junction 88) -> (junction 124) [order 1] : [AEBJunc_SameTarget == false]
  (junction 88) -> (junction 94) [order 2] : {
      | TOS_AEBJunc_TargetsDx = Object_Dx;
      | }
  (junction 124) -> (junction 114)
  (junction 114) -> (junction 117) [order 1] : [abs(Object_Vy) > P_TOS_AEBJuncTargetVyvThre_val ]
  (junction 114) -> (junction 118) [order 2] : {
      | TOS_AEBJunc_TargetsDx = single(255);
      | }
  (junction 117) -> (junction 112) : {
      | TOS_AEBJunc_TargetsDx = Object_Dx;
      | }
  (junction 112) -> (junction 118)
  (junction 118) -> (junction 125)
  (junction 94) -> (junction 97)
  (junction 125) -> (junction 94)
  (junction 97) -> (junction 100)
  data: AEBJunc_TargetCondition input boolean; Object_ID input uint8; psiDtOpt input single; AEBJunc_Target_ObjectID_K1 input uint8 size=32; Object_Vy input single; TOS_AEBJunc_TargetsDx output single size=1; Object_Dx input single; AEBJunc_SameTarget local boolean size=1 =false; P_TOS_AEBJuncTargetVyvThre_val parameter; P_TOS_AEBJuncTargetEgoYawRateThre_val parameter; C_TOS_AEBJuncPedTargetSize_Val parameter

== stateflow chart PubIfDecisionTOS_MDL/TOS_20201112/TOS_2012080320/TOS/AEB/TOS_AEBJunct1105/AEBJunc_Object_Condition/AEBJA_TargetCondition/TOS_AEBJunc_TargetsCondition/AEBJunc_VehTargetCondition/Chart ==
  state AEBJuncSameTargetIDJudge [function]
    (default) -> (junction 70) : {
        | i = uint8(1);
        | AEBJunc_SameTarget = false;
        | }
    (junction 70) -> (junction 81) [order 1] : [i<=C_TOS_AEBJuncPedTargetSize_Val]
    (junction 86) -> (junction 70)
    (junction 70) -> (junction 83) [order 2]
    (junction 81) -> (junction 77)
    (junction 77) -> (junction 78) [order 1] : [AEBJunc_Target_ObjectID_K1(i) == Object_ID]
    (junction 77) -> (junction 74) [order 2] : %donothing
    (junction 78) -> (junction 72) : {
        | AEBJunc_SameTarget = true;
        | }
    (junction 72) -> (junction 74)
    (junction 74) -> (junction 86) : {i = i+1;}
  (default) -> (junction 1)
  (junction 1) -> (junction 3) [order 1] : [AEBJunc_TargetCondition == true]
  (junction 1) -> (junction 97) [order 2] : {
      | TOS_AEBJunc_TargetsDx = single(255);
      | }
  (junction 3) -> (junction 88) : {
      | AEBJuncSameTargetIDJudge();
      | }
  (junction 88) -> (junction 124) [order 1] : [AEBJunc_SameTarget == false]
  (junction 88) -> (junction 94) [order 2] : {
      | TOS_AEBJunc_TargetsDx = Object_Dx;
      | }
  (junction 124) -> (junction 114)
  (junction 114) -> (junction 117) [order 1] : [abs(Object_Vy) > P_TOS_AEBJuncTargetVyvThre_val &&...
      | abs(psiDtOpt) < P_TOS_AEBJuncTargetEgoYawRateThre_val]
  (junction 114) -> (junction 118) [order 2] : {
      | TOS_AEBJunc_TargetsDx = single(255);
      | }
  (junction 117) -> (junction 112) : {
      | TOS_AEBJunc_TargetsDx = Object_Dx;
      | }
  (junction 112) -> (junction 118)
  (junction 118) -> (junction 125)
  (junction 94) -> (junction 97)
  (junction 125) -> (junction 94)
  (junction 97) -> (junction 100)
  data: AEBJunc_TargetCondition input boolean; Object_ID input uint8; psiDtOpt input single; AEBJunc_Target_ObjectID_K1 input uint8 size=32; Object_Vy input single; TOS_AEBJunc_TargetsDx output single size=1; Object_Dx input single; AEBJunc_SameTarget local boolean size=1 =false; P_TOS_AEBJuncTargetVyvThre_val parameter; P_TOS_AEBJuncTargetEgoYawRateThre_val parameter; C_TOS_AEBJuncPedTargetSize_Val parameter

== stateflow chart PubIfDecisionTOS_MDL/TOS_20201112/TOS_2012080320/TOS/AEB/TOS_AEBJunct1105/AEBJunc_Object_Condition1/AEBJA_TargetCondition/TOS_AEBJunc_TargetsCondition/AEBJunc_PedTargetCondition/Chart ==
  state AEBJuncSameTargetIDJudge [function]
    (default) -> (junction 70) : {
        | i = uint8(1);
        | AEBJunc_SameTarget = false;
        | }
    (junction 70) -> (junction 81) [order 1] : [i<=C_TOS_AEBJuncPedTargetSize_Val]
    (junction 86) -> (junction 70)
    (junction 70) -> (junction 83) [order 2]
    (junction 81) -> (junction 77)
    (junction 77) -> (junction 78) [order 1] : [AEBJunc_Target_ObjectID_K1(i) == Object_ID]
    (junction 77) -> (junction 74) [order 2] : %donothing
    (junction 78) -> (junction 72) : {
        | AEBJunc_SameTarget = true;
        | }
    (junction 72) -> (junction 74)
    (junction 74) -> (junction 86) : {i = i+1;}
  (default) -> (junction 1)
  (junction 1) -> (junction 3) [order 1] : [AEBJunc_TargetCondition == true]
  (junction 1) -> (junction 97) [order 2] : {
      | TOS_AEBJunc_TargetsDx = single(255);
      | }
  (junction 3) -> (junction 88) : {
      | AEBJuncSameTargetIDJudge();
      | }
  (junction 88) -> (junction 124) [order 1] : [AEBJunc_SameTarget == false]
  (junction 88) -> (junction 94) [order 2] : {
      | TOS_AEBJunc_TargetsDx = Object_Dx;
      | }
  (junction 124) -> (junction 114)
  (junction 114) -> (junction 117) [order 1] : [abs(Object_Vy) > P_TOS_AEBJuncTargetVyvThre_val &&...
      | abs(psiDtOpt) < P_TOS_AEBJuncTargetEgoYawRateThre_val]
  (junction 114) -> (junction 118) [order 2] : {
      | TOS_AEBJunc_TargetsDx = single(255);
      | }
  (junction 117) -> (junction 112) : {
      | TOS_AEBJunc_TargetsDx = Object_Dx;
      | }
  (junction 112) -> (junction 118)
  (junction 118) -> (junction 125)
  (junction 94) -> (junction 97)
  (junction 125) -> (junction 94)
  (junction 97) -> (junction 100)
  data: AEBJunc_TargetCondition input boolean; Object_ID input uint8; psiDtOpt input single; AEBJunc_Target_ObjectID_K1 input uint8 size=32; Object_Vy input single; TOS_AEBJunc_TargetsDx output single size=1; Object_Dx input single; AEBJunc_SameTarget local boolean size=1 =false; P_TOS_AEBJuncTargetVyvThre_val parameter; P_TOS_AEBJuncTargetEgoYawRateThre_val parameter; C_TOS_AEBJuncPedTargetSize_Val parameter

== stateflow chart PubIfDecisionTOS_MDL/TOS_20201112/TOS_2012080320/TOS/AEB/TOS_AEBJunct1105/AEBJunc_Object_Condition1/AEBJA_TargetCondition/TOS_AEBJunc_TargetsCondition/AEBJunc_VehTargetCondition/Chart ==
  state AEBJuncSameTargetIDJudge [function]
    (default) -> (junction 70) : {
        | i = uint8(1);
        | AEBJunc_SameTarget = false;
        | }
    (junction 70) -> (junction 81) [order 1] : [i<=C_TOS_AEBJuncPedTargetSize_Val]
    (junction 86) -> (junction 70)
    (junction 70) -> (junction 83) [order 2]
    (junction 81) -> (junction 77)
    (junction 77) -> (junction 78) [order 1] : [AEBJunc_Target_ObjectID_K1(i) == Object_ID]
    (junction 77) -> (junction 74) [order 2] : %donothing
    (junction 78) -> (junction 72) : {
        | AEBJunc_SameTarget = true;
        | }
    (junction 72) -> (junction 74)
    (junction 74) -> (junction 86) : {i = i+1;}
  (default) -> (junction 1)
  (junction 1) -> (junction 3) [order 1] : [AEBJunc_TargetCondition == true]
  (junction 1) -> (junction 97) [order 2] : {
      | TOS_AEBJunc_TargetsDx = single(255);
      | }
  (junction 3) -> (junction 88) : {
      | AEBJuncSameTargetIDJudge();
      | }
  (junction 88) -> (junction 124) [order 1] : [AEBJunc_SameTarget == false]
  (junction 88) -> (junction 94) [order 2] : {
      | TOS_AEBJunc_TargetsDx = Object_Dx;
      | }
  (junction 124) -> (junction 114)
  (junction 114) -> (junction 117) [order 1] : [abs(Object_Vy) > P_TOS_AEBJuncTargetVyvThre_val &&...
      | abs(psiDtOpt) < P_TOS_AEBJuncTargetEgoYawRateThre_val]
  (junction 114) -> (junction 118) [order 2] : {
      | TOS_AEBJunc_TargetsDx = single(255);
      | }
  (junction 117) -> (junction 112) : {
      | TOS_AEBJunc_TargetsDx = Object_Dx;
      | }
  (junction 112) -> (junction 118)
  (junction 118) -> (junction 125)
  (junction 94) -> (junction 97)
  (junction 125) -> (junction 94)
  (junction 97) -> (junction 100)
  data: AEBJunc_TargetCondition input boolean; Object_ID input uint8; psiDtOpt input single; AEBJunc_Target_ObjectID_K1 input uint8 size=32; Object_Vy input single; TOS_AEBJunc_TargetsDx output single size=1; Object_Dx input single; AEBJunc_SameTarget local boolean size=1 =false; P_TOS_AEBJuncTargetVyvThre_val parameter; P_TOS_AEBJuncTargetEgoYawRateThre_val parameter; C_TOS_AEBJuncPedTargetSize_Val parameter

== stateflow chart PubIfDecisionTOS_MDL/TOS_20201112/TOS_2012080320/TOS/AEB/TOS_AEBJunct1105/AEBJunctionTargetInfor/AEBJuncTargetObjectType/AEBJuncTargetObjectType/TOS_AEBJunc_TargetObjectType ==
  state AEBJuncSameTargetType [function]
    (default) -> (junction 39) : {
        | i = uint8(1);
        | AEBJunc_TargetObjectType = OFM_OBJ_TYPE_E.INVALID;
        | }
    (junction 39) -> (junction 40) [order 1] : [i<=C_TOS_AEBJATargetSize_Val]
    (junction 45) -> (junction 39)
    (junction 39) -> (junction 46) [order 2]
    (junction 40) -> (junction 41)
    (junction 41) -> (junction 42) [order 1] : [AEBJunc_Target_ObjectID_K1(i) == Object_ID]
    (junction 41) -> (junction 43) [order 2] : %donothing
    (junction 42) -> (junction 44) : {
        | AEBJunc_TargetObjectType = AEBJunc_Target_ObjectType_K1(i);
        | i = C_TOS_AEBJATargetSize_Val+uint8(1);
        | }
    (junction 44) -> (junction 43)
    (junction 43) -> (junction 45) : {i = i+uint8(1);}
  (default) -> (junction 1)
  (junction 1) -> (junction 5) [order 1] : [ObjectType == OFM_OBJ_TYPE_E.PEDESTRIAN||...
      | ObjectType == OFM_OBJ_TYPE_E.BICYCLE||...
      | ObjectType == OFM_OBJ_TYPE_E.MOTORBIKE||...
      | ObjectType == OFM_OBJ_TYPE_E.CAR||...
      | ObjectType == OFM_OBJ_TYPE_E.TRUCK]
  (junction 1) -> (junction 27) [order 2] : {
      | AEBJuncSameTargetType();
      | }
  (junction 5) -> (junction 26) : {
      | AEBJunc_TargetObjectType = ObjectType;
      | }
  (junction 26) -> (junction 27)
  (junction 27) -> (junction 30)
  data: ObjectType input Enum: OFM_OBJ_TYPE_E size=1; Object_ID input uint8 size=1; AEBJunc_Target_ObjectType_K1 input Enum: OFM_OBJ_TYPE_E size=32; AEBJunc_Target_ObjectID_K1 input uint8 size=32; AEBJunc_TargetObjectType output Enum: OFM_OBJ_TYPE_E size=1; C_TOS_AEBJATargetSize_Val parameter
